simulink model "Cholesky_Ex1"  (R2025a)
settings: Solver=VariableStepAuto  StartTime=0.0  StopTime=10  RelTol=1e-3
InitFcn:
  | A = single(rand(8,8));
undefined symbols (not defined in the file): S, static_input_Convolution_Stream_Ex1, Subsystem, vsva2197, xcvc1902
libraries: aieSolver x1, aieUtilities x1, vmcUtilities x1
settings Model: Creator=sdegala  LastModifiedBy=sdegala
settings ModelReferenceCC: EnableRefExpFcnMdlSchedulingChecks=on
settings RTWCC: GPUComputeCapability=3.5

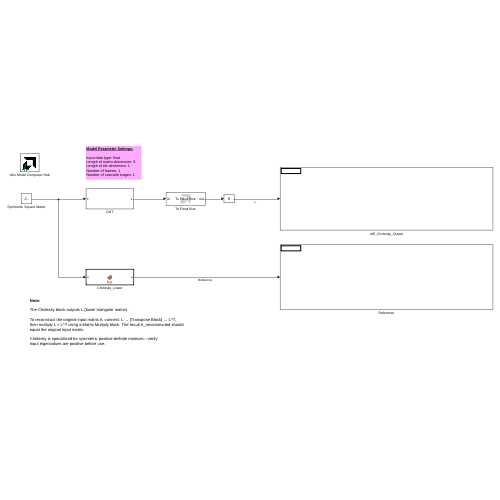
[thumbnail: Simulink's stored preview of the top-level diagram]
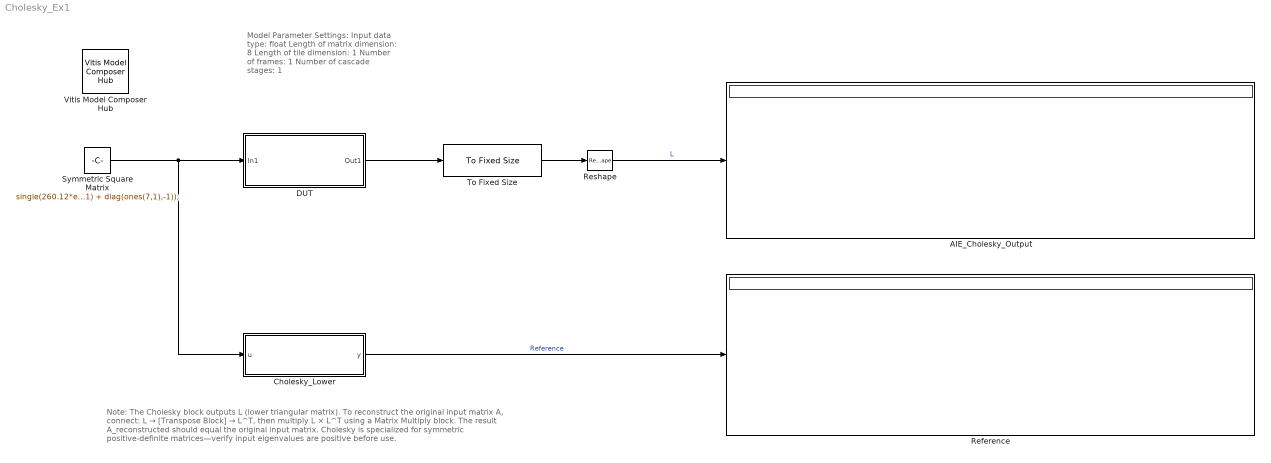
== system Cholesky_Ex1 ==
  note: Note:
      |
      | The Cholesky block outputs L (lower triangular matrix).
      |
      | To reconstruct the original input matrix A, connect: L → [Transpose Block] → L^T,
      | then multiply L × L^T using a Matrix Multiply block. The result A_reconstructed should
      | equal the original input matrix.
      |
      | Cholesky is specialized for symmetric positive-definite matrices—verify
      | input eigenvalues are positive before use.
  note: Model Parameter Settings:
      |
      | Input data type: float
      | Length of matrix dimension: 8
      | Length of tile dimension: 1
      | Number of frames: 1
      | Number of cascade stages: 1
  AIE_Cholesky_Output : Display
  Cholesky_Lower : MATLAB Function  TreatAsAtomicUnit=on
  DUT : Subsystem
  Reference : Display
  Reshape : Reshape  OutputDimensionality=Customize  OutputDimensions=[8,8]
  Symmetric Square Matrix : Constant  Value=single(260.12*eye(8) + diag(ones(7,1),1) + diag(ones(7,1),-1));  OutDataTypeStr=single  SampleTime=1
  To Fixed Size : aieUtilities/To Fixed Size  Mode=Stop simulation when input variable-size signal is not full  OutputSize=Inherit: Same as input  CopyMethod=Buffer samples to form output  HasStatusOutput=on
  Vitis Model Composer Hub : vmcUtilities/Vitis Model Composer Hub  Tag=genX  CodeGeneration=off  SubsystemName=Subsystem  BlockHierPath=static_input_Convolution_Stream_Ex1/Subsystem  SubsystemType=AIENode  AIEArrayConfig=Use entire AIE array  StartColumn=1  NumberOfColumns=1  TargetDirectory=./code  exportDesign=on  analyzeDesign=off  validateDesignOnHw=off  ExportType=AI Engines  IpVendor=xilinx.com  IpLibrary=hls  IpVersion=1.0  IpHWLanguage=Verilog  AieCompilerOptions={}  AieSimulatorOptions={}  CreateTestbench=on  TestbenchStackSize=10  RunRtlSim=off  RunCSim=off  RunAieSim=off  enableSimulationTimeout=on  enableGraphIterations=on  AieSimTimeout=50000  AieGraphIterations=-1  RunAieSimProfiling=off  LaunchVitisAnalyzer=off  PlotOutput=off  RunX86Sim=off  X86SimTimeout=10  GenHwImage=off  GenLibadfXo=off  GenHwValidationCode=off  PlatformType=Not Specified  HwSystemType=Baremetal  HwValidationTarget=hw  ProjDevice=xcvc1902-vsva2197-1LP-e-S  ProjDevicePart=xcvc1902-vsva2197-1LP-e-S  AIEType=AIE  SamplePeriod=-1  ClockFrequency=200  DataPathParallelism=1  xilinxfamily=versalaicore  part=xcvc1902  speed=-1LP-e-S  package=vsva2197  directory=./netlist  testbench=off  incr_netlist=off  synthesis_tool=Vivado  clock_wrapper=Clock Enables  dbl_ovrd=According to Block Masks  dcm_input_clock_period=10  sysclk_period=10  simulink_period=1  eval_field=0  IPInfoJsonString="{\"DUTSubsystemName\":\"Subsystem\",\"AIESubsystem\":{\"SubsystemName\":\"Subsystem\",\"TargetDirectory\":\"./code\",\"AIEArrayConfig\":\"Use entire AIE array\",\"StartColumn\":\"0\",\"NumberOfColumns\":\"1\"},\"SubsystemTag\":\"AIENode\"}"  LogFileName=/tmp/CR-1250814/code/model_composer.log  NThreads=4  IPConfigFile=/tmp/vmctmp-13380004059271250980/static_input_Convolution_Stream_Ex1_ipconfig.json
  wires:
  Symmetric Square Matrix/1 -> DUT/1(In1), Cholesky_Lower/1(u)
  To Fixed Size/1 -> Reshape/1
  Cholesky_Lower/1(y) -> Reference/1  "Reference"
  Reshape/1 -> AIE_Cholesky_Output/1  "L"
  DUT/1(Out1) -> To Fixed Size/1

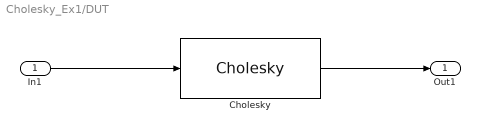
== system Cholesky_Ex1/DUT ==
  In1 : Inport
  Cholesky : aieSolver/Cholesky  AIE_VARIANT=1  data_type=float  dim_matrix=8  grid_dimension=1  num_frames=1  casc_length=1  inversion_diag=off  blockJsonConstraints=[]  blockJsonConstraintsInternal=[]  spec=vmc_cholesky.json  SerializedMaskParamNames=[]  SerializedMaskParamValues=[]  SerializedMaskParamVisibilities=[]  block_type=Cholesky  SerializedMaskParamDataypes=uint|typename|uint|uint|uint|uint|uint  SerializedMaskParamEnumStrArr=0|0|0|0|0|0|0  SerializedMaskParamEnumValArr=0|0|0|0|0|0|0  SerializedMaskParamVectorArr=0|0|0|0|0|0|0  SerializedMaskParamKeys=AIE_VARIANT|TT_DATA|TP_DIM|TP_GRID_DIM|TP_NUM_FRAMES|TP_CASC_LEN|TP_DIAG_INV
  Out1 : Outport
  wires:
  Cholesky/1 -> Out1/1
  In1/1 -> Cholesky/1

== matlab function Cholesky_Ex1/Cholesky_Lower ==
  data: u input; y output
function y = fcn(u)

y = single(chol(u,'lower'));
